simulink model "ukf_cfg0"  (R2013b)
settings: Solver=FixedStepDiscrete  StartTime=0.0  StopTime=59  FixedStep=0.1  RelTol=1e-3
InitFcn:
  | clear all; ukf
settings Model: PauseTimes=93.4  SnapshotBufferSize=5  SnapshotInterval=5  Creator=igeorgie  LastModifiedBy=igeorgie

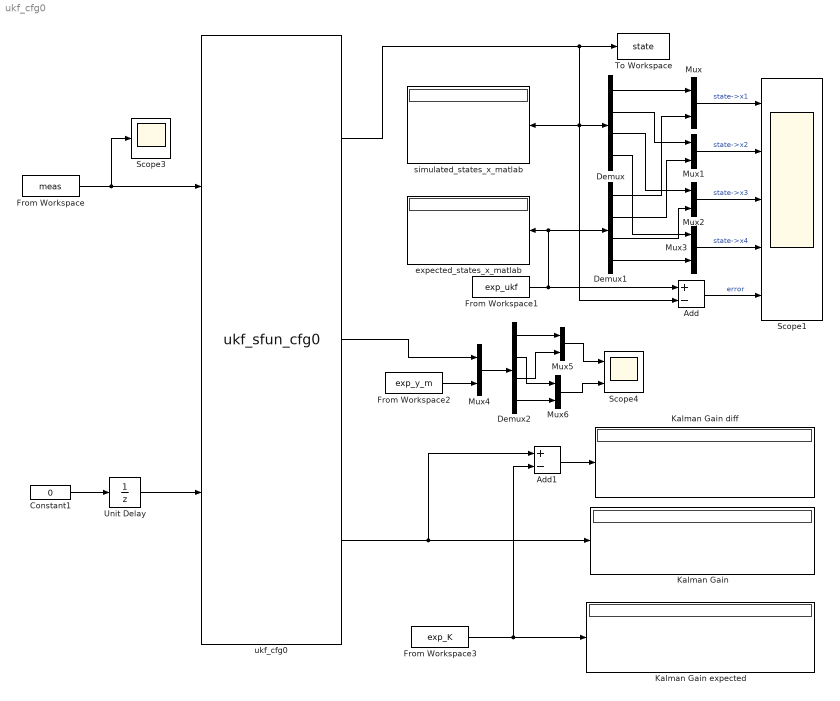
== system ukf_cfg0 ==
  Add : Sum  Inputs=+-
  Add1 : Sum  Inputs=+-
  Constant1 : Constant  Value=0  OutDataTypeStr=double  SampleTime=0.1
  Demux : Demux
  Demux1 : Demux
  Demux2 : Demux
  From Workspace : FromWorkspace  VariableName=meas  SampleTime=0.1  Interpolate=off  OutputAfterFinalValue=Holding final value
  From Workspace1 : FromWorkspace  VariableName=exp_ukf  SampleTime=0.1  Interpolate=off  OutputAfterFinalValue=Holding final value
  From Workspace2 : FromWorkspace  VariableName=exp_y_m  SampleTime=0.1  Interpolate=off  OutputAfterFinalValue=Holding final value
  From Workspace3 : FromWorkspace  VariableName=exp_K  SampleTime=0.1  Interpolate=off  OutputAfterFinalValue=Holding final value
  Kalman Gain : Display
  Kalman Gain diff : Display
  Kalman Gain expected : Display
  Mux{,1..6} (7 alike) : Mux  Inputs=2
  Scope1 : Scope  NumInputPorts=5
      settings: TickLabels=on  YMin=-5~-5~-5~-5~-5  YMax=5~5~5~5~5
  Scope3 : Scope
      settings: SaveName=ScopeData2
  Scope4 : Scope  NumInputPorts=2
      settings: YMin=-5~-5  YMax=5~5  SaveName=ScopeData3
  To Workspace : ToWorkspace  VariableName=state  SampleTime=-1
  Unit Delay : UnitDelay  InitialCondition=1  SampleTime=0.1
  expected_states_x_matlab : Display
  simulated_states_x_matlab : Display
  ukf_cfg0 : S-Function  InitFcn=try, set_param(gcb,'FunctionName','ukf_sfun_cfg0'), end  FunctionName=ukf_sfun_cfg0  SFunctionModules=ukf_sfun_cfg0_wrapper ukfLib mtxLib ukfCfg ukfCfg1  EnableBusSupport=off  mask(S-Function Builder){}
      mask help: Simulink:masks:SFunctionBuilder_MD
      mask init:
      | val = [[.9  0.75 0.75 1 1 .9 .9 1]',[1 1 0.75 0.75 .9 .9 1 .9]'];try , sys = get_param(gcb,'SfunBuilderFcnName');if isempty(sys), sys = get_param(gcb,'FunctionName'); end,catch, sys = get_param(gcb,'FunctionName'); end
      settings: CopyFcn=set_param(gcbh,'LinkStatus','none')  PreSaveFcn=try, set_param(gcb,'FunctionName','ukf_sfun_cfg0'), end  OpenFcn=sfunctionwizard(gcbh)
      mask Display: plot(val(:,1),val(:,2)),disp(sys), port_label('input',1,'meas'), port_label('input',2,'Init'), port_label('output',1,'states'), port_label('output',2,'y_mean'), port_label('output',3,'kalman')
  wires:
  ukf_cfg0/2 -> Mux4/1
  Unit Delay/1 -> ukf_cfg0/2
  Constant1/1 -> Unit Delay/1
  From Workspace/1 -> ukf_cfg0/1, Scope3/1
  From Workspace1/1 -> expected_states_x_matlab/1, Demux1/1, Add/1
  Mux/1 -> Scope1/1  "state->x1"
  Demux/1 -> Mux/1
  Demux1/1 -> Mux/2
  Mux1/1 -> Scope1/2  "state->x2"
  Demux/2 -> Mux1/1
  Demux1/2 -> Mux1/2
  Demux/3 -> Mux2/1
  Demux1/3 -> Mux2/2
  Mux2/1 -> Scope1/3  "state->x3"
  Demux/4 -> Mux3/1
  Demux1/4 -> Mux3/2
  Mux3/1 -> Scope1/4  "state->x4"
  ukf_cfg0/1 -> Demux/1, Add/2, simulated_states_x_matlab/1, To Workspace/1
  Add/1 -> Scope1/5  "error"
  ukf_cfg0/3 -> Add1/1, Kalman Gain/1
  From Workspace2/1 -> Mux4/2
  Mux4/1 -> Demux2/1
  Demux2/1 -> Mux5/1
  Demux2/3 -> Mux5/2
  Demux2/2 -> Mux6/1
  Demux2/4 -> Mux6/2
  Mux5/1 -> Scope4/1
  Mux6/1 -> Scope4/2
  From Workspace3/1 -> Add1/2, Kalman Gain expected/1
  Add1/1 -> Kalman Gain diff/1
